simulink model "final_3_20250707"  (R2021a)
settings: Solver=ode4  StartTime=0.0  StopTime=100  FixedStep=0.0001  RelTol=1e-3
values from neighbouring files (symbols this model uses):
  tita = 4    [final_1_20250707.m]
  ue = x2e    [final_1_20250707.m]
  x1e = 20    [final_1_20250707.m]
  x2e = (m*(g*sind(tita)+g*C_r+(1/(2*m))*ro*C_d*A_var*x1e^2))/(alfa_n*T_m*(1-beta*(((alfa_n*x1e)/w_m)-1)^2))    [final_1_20250707.m]
  x3e = 0    [final_1_20250707.m]
  ye = x1e    (= 20)    [final_1_20250707.m]
libraries: cstblocks x2
settings Model: Creator=aghersin  LastModifiedBy=frand
settings SolverCC: AlgebraicLoopSolver=TrustRegion
settings DataIOCC: ReturnWorkspaceOutputs=off
settings OptimizationCC: LifeSpan=inf
settings DebuggingCC: SFExecutionAtInitializationDiag=none  SFMachineParentedDataDiag=warning  ArithmeticOperatorsInVariantConditions=warning
settings SFSimCC: SimUseLocalCustomCode=off  CustomCodeUndefinedFunction=UseInterfaceOnly
settings RTWCC: RTWUseLocalCustomCode=off
settings CodeAppCC: StateflowObjectComments=on

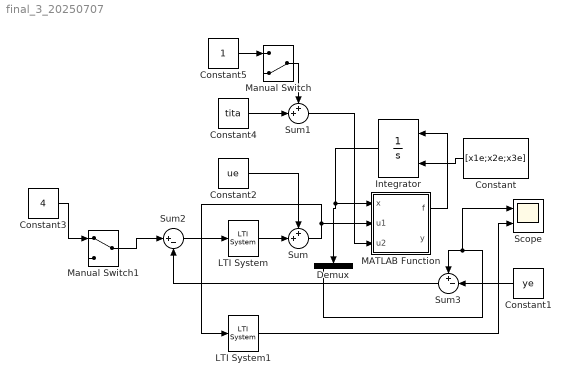
== system final_3_20250707 ==
  Constant : Constant  Value=[x1e;x2e;x3e]
  Constant1 : Constant  Value=ye
  Constant2 : Constant  Value=ue
  Constant3 : Constant  Value=4
  Constant4 : Constant  Value=tita
  Constant5 : Constant
  Demux : Demux  Outputs=3
  Integrator : Integrator  InitialConditionSource=external
  LTI System : cstblocks/LTI System  sys=C_dig  IC=[]
  LTI System1 : cstblocks/LTI System  sys=U_u  IC=[]
  MATLAB Function : MATLAB Function  TreatAsAtomicUnit=on
  Manual Switch : ManualSwitch  CurrentSetting=0
  Manual Switch1 : ManualSwitch
  Scope : Scope  NumInputPorts=2
  Sum : Sum  Inputs=++|
  Sum1 : Sum  Inputs=++|
  Sum2 : Sum  Inputs=|+-
  Sum3 : Sum  Inputs=+-|
  wires:
  Integrator/1 -> Demux/1, MATLAB Function/1(x)
  MATLAB Function/1(f) -> Integrator/1
  Constant/1 -> Integrator/2
  Constant1/1 -> Sum3/2
  Constant2/1 -> Sum/1
  Sum2/1 -> LTI System/1
  Sum3/1 -> Sum2/2
  LTI System/1 -> Sum/2
  Sum/1 -> LTI System1/1, MATLAB Function/2(u1)
  Demux/1 -> Scope/1, Sum3/1
  LTI System1/1 -> Scope/2
  Constant4/1 -> Sum1/2
  Sum1/1 -> MATLAB Function/3(u2)
  Constant3/1 -> Manual Switch1/1
  Manual Switch1/1 -> Sum2/1
  Constant5/1 -> Manual Switch/1
  Manual Switch/1 -> Sum1/1

== matlab function final_3_20250707/MATLAB Function ==
  data: x input; u1 input; f output; y output; u2 input
function [f,y] = fcn(x,u1,u2)

m = 1600;
T_m = 190;
w_m = 420;
beta = 0.4;
g = 9.8;
C_r = 0.01;
ro = 1.3;
C_d = 0.32;
A_var = 2.4;
alfa_n = 12;
w_n = 2*pi;


f1 = (alfa_n/m)*x(2)*T_m*(1-beta*((alfa_n*x(1))/w_m)^2)-g*sind(u2)+g*C_r+(1/(2*m))*ro*C_d*A_var*x(1)^2;

f2 = x(3);

f3 = (w_n)^2*u1-2*w_n*x(3)-(w_n)^2*x(2);

f=[f1;f2;f3];

y=x(1);
